simulink subsystem "DIEC"  (R2024a)
settings: Solver=VariableStepAuto  StartTime=0.0  StopTime=10.0  RelTol=1e-3
settings Model: Creator=prony  LastModifiedBy=nicol

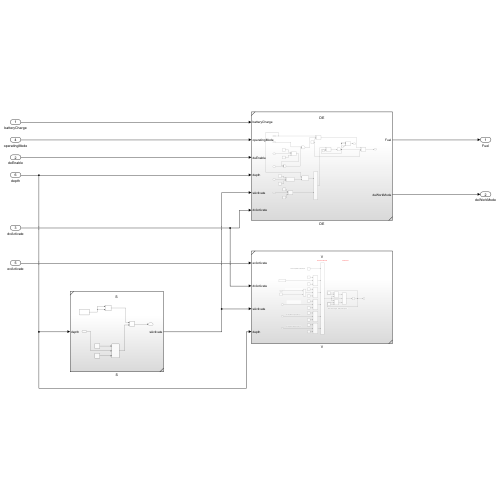
[thumbnail: Simulink's stored preview of the top-level diagram]
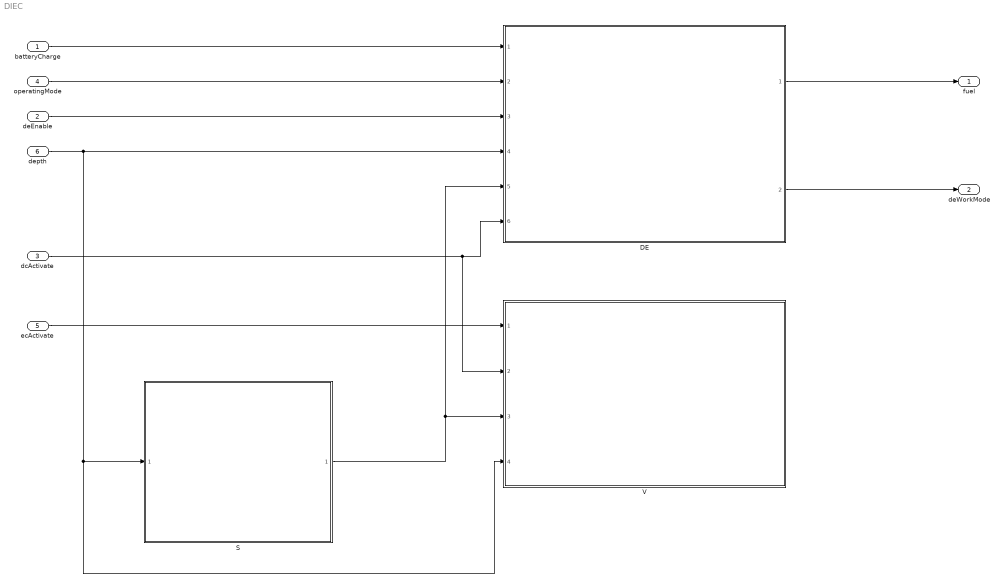
== system DIEC ==
  batteryCharge : Inport
  deEnable : Inport  Port=2
  dcActivate : Inport  Port=3
  operatingMode : Inport  Port=4
  ecActivate : Inport  Port=5
  depth : Inport  Port=6
  DE : Subsystem  ReferencedSubsystem=DE
  S : Subsystem  ReferencedSubsystem=S
  V : Subsystem  ReferencedSubsystem=V
  fuel : Outport
  deWorkMode : Outport  Port=2
  wires:
  batteryCharge/1 -> DE/1
  deEnable/1 -> DE/3
  operatingMode/1 -> DE/2
  S/1 -> V/3, DE/5
  dcActivate/1 -> V/2, DE/6
  ecActivate/1 -> V/1
  DE/2 -> deWorkMode/1
  DE/1 -> fuel/1
  depth/1 -> DE/4, V/4, S/1
